simulink model "SF042A_HwAgSnsrls"  (R2013b)
settings: Solver=FixedStepDiscrete  SolverMode=SingleTasking  StartTime=0.0  StopTime=1  FixedStep=0.002  RelTol=1e-3
values from neighbouring files (symbols this model uses):
  ARCHGLBPRM_2MILLISEC_SEC_F32 = DataDict.Constant    [SF042A_HwAgSnsrls_DataDict.m]
  CORRDPINIONAGCON_CNT_U08 = DataDict.Constant    [SF042A_HwAgSnsrls_DataDict.m]
  FCENTROFFSCON_CNT_U08 = DataDict.Constant    [SF042A_HwAgSnsrls_DataDict.m]
  HwAgSnsrlsCorrdPinionAgHwConf = DataDict.Calibration    [SF042A_HwAgSnsrls_DataDict.m]
  HwAgSnsrlsFCentrHwConf = DataDict.Calibration    [SF042A_HwAgSnsrls_DataDict.m]
  HwAgSnsrlsSmotngCoeff = DataDict.Calibration    [SF042A_HwAgSnsrls_DataDict.m]
  HwAgSnsrlsSmotngStepThd = DataDict.Calibration    [SF042A_HwAgSnsrls_DataDict.m]
  HwAgSnsrlsStordPinionConf = DataDict.Calibration    [SF042A_HwAgSnsrls_DataDict.m]
  HwAgSnsrlsStordPinionConfThd = DataDict.Calibration    [SF042A_HwAgSnsrls_DataDict.m]
  HwAgSnsrlsVehDynDifThd = DataDict.Calibration    [SF042A_HwAgSnsrls_DataDict.m]
  HwAgSnsrlsVehDynHwConf = DataDict.Calibration    [SF042A_HwAgSnsrls_DataDict.m]
  HwAgSnsrlsVehDynMotVelThd = DataDict.Calibration    [SF042A_HwAgSnsrls_DataDict.m]
  HwAgSnsrlsVehDynPinionTqThd = DataDict.Calibration    [SF042A_HwAgSnsrls_DataDict.m]
  HwAgSnsrlsVehDynTmr1Thd = DataDict.Calibration    [SF042A_HwAgSnsrls_DataDict.m]
  HwAgSnsrlsVehDynTmr2Thd = DataDict.Calibration    [SF042A_HwAgSnsrls_DataDict.m]
  HwAgSnsrlsVehDynVehSpdThd = DataDict.Calibration    [SF042A_HwAgSnsrls_DataDict.m]
  HwAgSnsrlsVehDynYawRateThd = DataDict.Calibration    [SF042A_HwAgSnsrls_DataDict.m]
  HwAgSnsrlsWhlFrqThd = DataDict.Calibration    [SF042A_HwAgSnsrls_DataDict.m]
  HwAgSnsrlsWhlSpdHwAgCoeff1 = DataDict.Calibration    [SF042A_HwAgSnsrls_DataDict.m]
  HwAgSnsrlsWhlSpdHwAgCoeff2 = DataDict.Calibration    [SF042A_HwAgSnsrls_DataDict.m]
  HwAgSnsrlsWhlSpdHwAgThd = DataDict.Calibration    [SF042A_HwAgSnsrls_DataDict.m]
  HwAgSnsrlsWhlSpdHwConf = DataDict.Calibration    [SF042A_HwAgSnsrls_DataDict.m]
  HwAgSnsrlsWhlSpdRatThd = DataDict.Calibration    [SF042A_HwAgSnsrls_DataDict.m]
  HwAgSnsrlsWhlSpdTmrThd = DataDict.Calibration    [SF042A_HwAgSnsrls_DataDict.m]
  HwAgSnsrlsWhlSpdVehSpdThd = DataDict.Calibration    [SF042A_HwAgSnsrls_DataDict.m]
  LASTPOSNCON_CNT_U08 = DataDict.Constant    [SF042A_HwAgSnsrls_DataDict.m]
  MILLISECTO100MICROSEC_ULS_U32 = DataDict.Constant    [SF042A_HwAgSnsrls_DataDict.m]
  SysGlbPrmSysKineRat = DataDict.ImprtdCal    [SF042A_HwAgSnsrls_DataDict.m]
  SysGlbPrmSysTqRat = DataDict.ImprtdCal    [SF042A_HwAgSnsrls_DataDict.m]
  VEHDYNCON_CNT_U08 = DataDict.Constant    [SF042A_HwAgSnsrls_DataDict.m]
  WHLSPDCON_CNT_U08 = DataDict.Constant    [SF042A_HwAgSnsrls_DataDict.m]
undefined symbols (not defined in the file or in its folder): NtcNr1, SigQlfr1
libraries: NxtrAbslt x11, Fil x8, NxtrLim x4, simulink x3, NxtrNvM x1, FixdToFloat x1
(part 2 of 6)

== system SF042A_HwAgSnsrls/HwAgSnsrls/HwAgSnsrlsInit1/FiltersInit ==
  CopyRight2 : Subsystem  Description=|  mask(Copyright Information){none=on}
      | Copyright info block.                                               
      |                                                                     
      | Place copyright information at the top of every subsystem in design.
      mask prompts: none "No parameters"
      mask help: Place copyright information at the top of every subsystem in design.
      mask Display:
      | NxtrConf = 'Nexteer Confidential';
      | 
      | sys = bdroot; %handle for the current model ("system")
      | first = get_param(sys,'Created');
      | if(isempty(first))
      |     first = datestr(now,'yyyy');
      | else
      |     first = first(end-3:end);  %year is last four digits
      | end
      | 
      | last = get_param(sys,'LastModifiedDate');
      | if isempty(last)
      |     last = datestr(now,'yyyy');
      | else
      |     last = last(end-3:end);
      | end
      | 
      | if strcmp(first,last)
      |     fprintf('%s -- Copyright %s Nexteer',NxtrConf,first)
      | else
      |     fprintf('%s -- %s%s- %s Nexteer',NxtrConf,char(169),first,last)
      | end
  PinionTqFilInit : Fil/FilLpInit  Ic=0  Ts=ARCHGLBPRM_2MILLISEC_SEC_F32  Freq=HwAgSnsrlsPinionTqFilFrq  StVar=PinionTqFil
  RelHwAgFil1Init : Fil/FilLpInit  Ic=0  Ts=ARCHGLBPRM_2MILLISEC_SEC_F32  Freq=HwAgSnsrlsRelHwAgFil1Frq  StVar=RelHwAgFil1
  RelHwAgFil2Init : Fil/FilLpInit  Ic=0  Ts=ARCHGLBPRM_2MILLISEC_SEC_F32  Freq=HwAgSnsrlsRelHwAgFil2Frq  StVar=RelHwAgFil2
  YawRateFilInit : Fil/FilLpInit  Ic=0  Ts=ARCHGLBPRM_2MILLISEC_SEC_F32  Freq=HwAgSnsrlsYawRateFilFrq  StVar=YawRateFil

== system SF042A_HwAgSnsrls/HwAgSnsrls/HwAgSnsrlsInit1/GetNtcQlfrSts ==
  NtcNr : Inport
  CopyRight2 : Subsystem  Description=|  mask(Copyright Information){none=on}
      | Copyright info block.                                               
      |                                                                     
      | Place copyright information at the top of every subsystem in design.
      mask prompts: none "No parameters"
      mask help: Place copyright information at the top of every subsystem in design.
      mask Display:
      | NxtrConf = 'Nexteer Confidential';
      | 
      | sys = bdroot; %handle for the current model ("system")
      | first = get_param(sys,'Created');
      | first = first(end-3:end);  %year is last four digits
      | 
      | last = get_param(sys,'LastModifiedDate');
      | if isempty(last)
      |     last = datestr(now,'yyyy');
      | else
      |     last = last(end-3:end);
      | end
      | 
      | if strcmp(first,last)
      |     fprintf('%s -- Copyright %s Nexteer',NxtrConf,first)
      | else
      |     fprintf('%s -- %s%s- %s Nexteer',NxtrConf,char(169),first,last)
      | end
  Data Store Read : DataStoreRead  DataStoreName=NtcQlfr
  Terminator : Terminator
  NtcQlfr : Outport
  wires:
  Data Store Read/1 -> NtcQlfr/1
  NtcNr/1 -> Terminator/1

== system SF042A_HwAgSnsrls/HwAgSnsrls/HwAgSnsrlsInit1/GetRefTmr100MicroSec32bit ==
  note: Created Aug 18, 2015
      | Modified Oct 21, 2015
      | Modified Oct 30, 2015
      | Kevin Derry
  note: GetRefTmr100MicroSec32bit
  note: Wrap-to-zero
  note: counts
  note: microseconds
  note: seconds
  note: 1 count = 100 uSec
  CopyRight2 : Subsystem  Description=|  mask(Copyright Information){none=on}
      | Copyright info block.                                               
      |                                                                     
      | Place copyright information at the top of every subsystem in design.
      mask prompts: none "No parameters"
      mask help: Place copyright information at the top of every subsystem in design.
      mask Display:
      | NxtrConf = 'Nexteer Confidential';
      | 
      | sys = bdroot; %handle for the current model ("system")
      | first = get_param(sys,'Created');
      | if(isempty(first))
      |     first = datestr(now,'yyyy');
      | else
      |     first = first(end-3:end);  %year is last four digits
      | end
      | 
      | last = get_param(sys,'LastModifiedDate');
      | if isempty(last)
      |     last = datestr(now,'yyyy');
      | else
      |     last = last(end-3:end);
      | end
      | 
      | if strcmp(first,last)
      |     fprintf('%s -- Copyright %s Nexteer',NxtrConf,first)
      | else
      |     fprintf('%s -- %s%s- %s Nexteer',NxtrConf,char(169),first,last)
      | end
  Count per uSec : Constant  Value=0.01
  Data Store Read1 : DataStoreRead  DataStoreName=SimnTi
  Data Type Conversion1 : DataTypeConversion  OutDataTypeStr=uint32
  Divide1 : Product  Inputs=**
  Divide2 : Product  Inputs=*/
  Max Counts : Constant  Value=2^32-1
  Product1 : Product
  Product2 : Product
  Rounding : Rounding
  Subtract1 : Sum  Inputs=+-
  uSec per Sec : Constant  Value=1000000
  RefTmr : Outport
  wires:
  Data Store Read1/1 -> Product1/1
  Data Type Conversion1/1 -> RefTmr/1
  uSec per Sec/1 -> Product1/2
  Count per uSec/1 -> Divide1/2
  Product1/1 -> Divide1/1
  Divide1/1 -> Subtract1/1, Divide2/1
  Max Counts/1 -> Product2/2, Divide2/2
  Divide2/1 -> Rounding/1
  Rounding/1 -> Product2/1
  Subtract1/1 -> Data Type Conversion1/1
  Product2/1 -> Subtract1/2

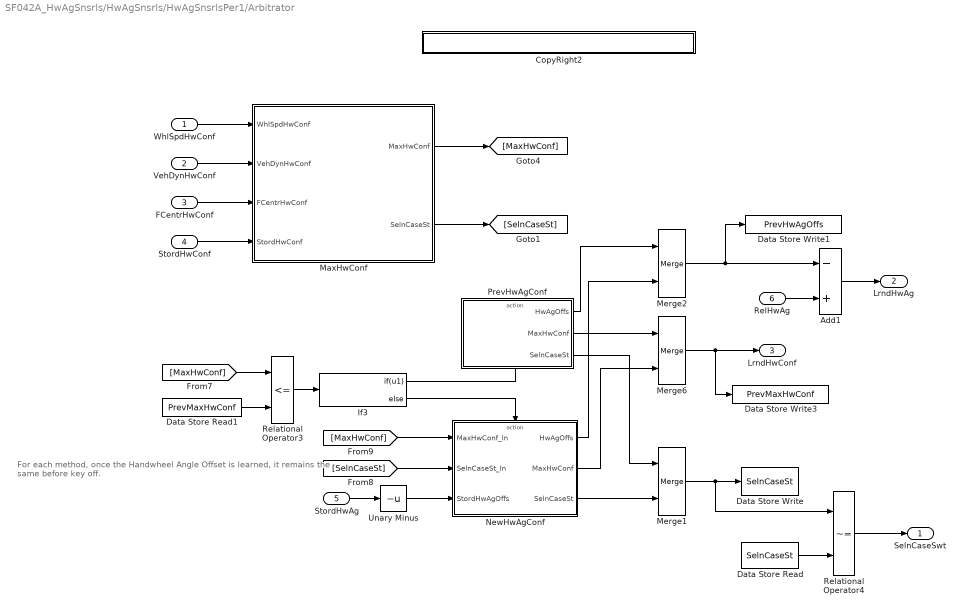
== system SF042A_HwAgSnsrls/HwAgSnsrls/HwAgSnsrlsPer1/Arbitrator ==
  note: For each method, once the Handwheel Angle Offset is learned, it remains the
      | same before key off.
  WhlSpdHwConf : Inport
  VehDynHwConf : Inport  Port=2
  FCentrHwConf : Inport  Port=3
  StordHwConf : Inport  Port=4
  StordHwAg : Inport  Port=5
  RelHwAg : Inport  Port=6
  Add1 : Sum  RequirementInfo="{'linktype_rmi_doors' '00012961 (/E-STEER Core/SubSystem Specifications/Application Functions - EA4/SF042A Handwheel Angle Sensorless)' '#SF042A_91' 'true' 'REQ:  SF042A_91' '' } %GIDa_1ccd16d5_cbcc_41e9_85e2_2e3643f02b11"  Inputs=-+
  CopyRight2 : Subsystem  Description=|  mask(Copyright Information){none=on}
      | Copyright info block.                                               
      |                                                                     
      | Place copyright information at the top of every subsystem in design.
      mask prompts: none "No parameters"
      mask help: Place copyright information at the top of every subsystem in design.
      mask Display:
      | NxtrConf = 'Nexteer Confidential';
      | 
      | sys = bdroot; %handle for the current model ("system")
      | first = get_param(sys,'Created');
      | if(isempty(first))
      |     first = datestr(now,'yyyy');
      | else
      |     first = first(end-3:end);  %year is last four digits
      | end
      | 
      | last = get_param(sys,'LastModifiedDate');
      | if isempty(last)
      |     last = datestr(now,'yyyy');
      | else
      |     last = last(end-3:end);
      | end
      | 
      | if strcmp(first,last)
      |     fprintf('%s -- Copyright %s Nexteer',NxtrConf,first)
      | else
      |     fprintf('%s -- %s%s- %s Nexteer',NxtrConf,char(169),first,last)
      | end
  Data Store Read : DataStoreRead  Priority=1  DataStoreName=SelnCaseSt
  Data Store Read1 : DataStoreRead  RequirementInfo={} %GIDa_f23f8d3d_c4da_4f79_957d_263e33d41729  DataStoreName=PrevMaxHwConf
  Data Store Write : DataStoreWrite  Priority=2  DataStoreName=SelnCaseSt
  Data Store Write1 : DataStoreWrite  DataStoreName=PrevHwAgOffs
  Data Store Write3 : DataStoreWrite  DataStoreName=PrevMaxHwConf
  If3 : If  RequirementInfo={'linktype_rmi_doors' '00012961 (/E-STEER Core/SubSystem Specifications/Application Functions - EA4/SF042A Handwheel Angle Sensorless)' '#SF042A_80' 'true' 'REQ:SF042A_80' '' ; 'linktype_rmi_doors' '00012961 (/E-STEER Core/SubSystem Specifications/Application Functions - EA4/SF042A Handwheel Angle Sensorless)' '#SF042A_90' 'true' 'REQ:SF042A_90' '' } %GIDa_130cdf60_6fef_48e9_8b09_d21ec738d534  IfExpression=u1
  MaxHwConf : Subsystem  RequirementInfo={'linktype_rmi_doors' '00012961 (/E-STEER Core/SubSystem Specifications/Application Functions - EA4/SF042A Handwheel Angle Sensorless)' '#SF042A_80' 'true' 'REQ:SF042A_80' '' } %GIDa_e5157a28_4abb_4275_9ef4_fab061bcf0ff
  Merge1 : Merge  RequirementInfo={'linktype_rmi_doors' '00012961 (/E-STEER Core/SubSystem Specifications/Application Functions - EA4/SF042A Handwheel Angle Sensorless)' '#SF042A_90' 'true' 'REQ:SF042A_90' '' ; 'linktype_rmi_doors' '00012961 (/E-STEER Core/SubSystem Specifications/Application Functions - EA4/SF042A Handwheel Angle Sensorless)' '#SF042A_80' 'true' 'REQ:SF042A_80' '' } %GIDa_5b272a3b_1995_4619_bc08_9d470fec44f3
  Merge2 : Merge  RequirementInfo={'linktype_rmi_doors' '00012961 (/E-STEER Core/SubSystem Specifications/Application Functions - EA4/SF042A Handwheel Angle Sensorless)' '#SF042A_90' 'true' 'REQ:SF042A_90' '' ; 'linktype_rmi_doors' '00012961 (/E-STEER Core/SubSystem Specifications/Application Functions - EA4/SF042A Handwheel Angle Sensorless)' '#SF042A_80' 'true' 'REQ:SF042A_80' '' } %GIDa_c0f8c842_a58b_4714_b1d4_ec4b723ea5b6
  Merge6 : Merge  RequirementInfo={'linktype_rmi_doors' '00012961 (/E-STEER Core/SubSystem Specifications/Application Functions - EA4/SF042A Handwheel Angle Sensorless)' '#SF042A_90' 'true' 'REQ:SF042A_90' '' ; 'linktype_rmi_doors' '00012961 (/E-STEER Core/SubSystem Specifications/Application Functions - EA4/SF042A Handwheel Angle Sensorless)' '#SF042A_80' 'true' 'REQ:SF042A_80' '' } %GIDa_12b5e5e2_09a6_4992_9385_b86d5bcd82fa
  NewHwAgConf : Subsystem  RequirementInfo={'linktype_rmi_doors' '00012961 (/E-STEER Core/SubSystem Specifications/Application Functions - EA4/SF042A Handwheel Angle Sensorless)' '#SF042A_80' 'true' 'REQ:SF042A_80' '' } %GIDa_82674b30_ff3b_4424_92dc_60f07d4aa3b1  TreatAsAtomicUnit=on
  PrevHwAgConf : Subsystem  RequirementInfo={'linktype_rmi_doors' '00012961 (/E-STEER Core/SubSystem Specifications/Application Functions - EA4/SF042A Handwheel Angle Sensorless)' '#SF042A_90' 'true' 'REQ:SF042A_90' '' } %GIDa_34576ddf_b2ec_4043_bac4_f5bd2e7329f0  TreatAsAtomicUnit=on
  Relational Operator3 : RelationalOperator  RequirementInfo={'linktype_rmi_doors' '00012961 (/E-STEER Core/SubSystem Specifications/Application Functions - EA4/SF042A Handwheel Angle Sensorless)' '#SF042A_80' 'true' 'REQ:SF042A_80' '' ; 'linktype_rmi_doors' '00012961 (/E-STEER Core/SubSystem Specifications/Application Functions - EA4/SF042A Handwheel Angle Sensorless)' '#SF042A_90' 'true' 'REQ:SF042A_90' '' } %GIDa_f55476d1_a2bc_48a5_a5ff_0b6ad56709cd  Operator=<=  OutDataTypeStr=boolean
  Relational Operator4 : RelationalOperator  RequirementInfo={'linktype_rmi_doors' '00012961 (/E-STEER Core/SubSystem Specifications/Application Functions - EA4/SF042A Handwheel Angle Sensorless)' '#SF042A_81' 'true' 'REQ: SF042A_81' '' } %GIDa_b2c97a21_2f99_417c_b86c_11bc5588197e  Operator=~=  OutDataTypeStr=boolean
  Unary Minus : UnaryMinus
  SelnCaseSwt : Outport
  LrndHwAg : Outport  Port=2
  LrndHwConf : Outport  Port=3
  wires:
  [MaxHwConf] -> Relational Operator3/1
  Data Store Read1/1 -> Relational Operator3/2
  Relational Operator3/1 -> If3/1
  If3/1 -> PrevHwAgConf/Action
  If3/2 -> NewHwAgConf/Action
  [SelnCaseSt] -> NewHwAgConf/2(SelnCaseSt_In)
  [MaxHwConf] -> NewHwAgConf/1(MaxHwConf_In)
  PrevHwAgConf/2(MaxHwConf) -> Merge6/1
  Merge6/1 -> Data Store Write3/1, LrndHwConf/1
  NewHwAgConf/2(MaxHwConf) -> Merge6/2
  StordHwAg/1 -> Unary Minus/1
  Unary Minus/1 -> NewHwAgConf/3(StordHwAgOffs)
  Merge2/1 -> Data Store Write1/1, Add1/1
  RelHwAg/1 -> Add1/2
  Add1/1 -> LrndHwAg/1
  WhlSpdHwConf/1 -> MaxHwConf/1(WhlSpdHwConf)
  VehDynHwConf/1 -> MaxHwConf/2(VehDynHwConf)
  FCentrHwConf/1 -> MaxHwConf/3(FCentrHwConf)
  StordHwConf/1 -> MaxHwConf/4(StordHwConf)
  MaxHwConf/1(MaxHwConf) -> [MaxHwConf]
  MaxHwConf/2(SelnCaseSt) -> [SelnCaseSt]
  Data Store Read/1 -> Relational Operator4/2
  Relational Operator4/1 -> SelnCaseSwt/1
  NewHwAgConf/3(SelnCaseSt) -> Merge1/2
  PrevHwAgConf/3(SelnCaseSt) -> Merge1/1
  Merge1/1 -> Data Store Write/1, Relational Operator4/1
  NewHwAgConf/1(HwAgOffs) -> Merge2/2
  PrevHwAgConf/1(HwAgOffs) -> Merge2/1

== system SF042A_HwAgSnsrls/HwAgSnsrls/HwAgSnsrlsPer1/Case Invalid ==
  Action Port : ActionPort  ActionType=else
  Constant= : Constant  Value=false  OutDataTypeStr=boolean
      settings: AttributesFormatString=%<OutDataTypeStr>
  Constant=1 : Constant  Value=0  OutDataTypeStr=single
      settings: AttributesFormatString=%<OutDataTypeStr>
  CopyRight2 : Subsystem  Description=|  mask(Copyright Information){none=on}
      | Copyright info block.                                               
      |                                                                     
      | Place copyright information at the top of every subsystem in design.
      mask prompts: none "No parameters"
      mask help: Place copyright information at the top of every subsystem in design.
      mask Display:
      | NxtrConf = 'Nexteer Confidential';
      | 
      | sys = bdroot; %handle for the current model ("system")
      | first = get_param(sys,'Created');
      | if(isempty(first))
      |     first = datestr(now,'yyyy');
      | else
      |     first = first(end-3:end);  %year is last four digits
      | end
      | 
      | last = get_param(sys,'LastModifiedDate');
      | if isempty(last)
      |     last = datestr(now,'yyyy');
      | else
      |     last = last(end-3:end);
      | end
      | 
      | if strcmp(first,last)
      |     fprintf('%s -- Copyright %s Nexteer',NxtrConf,first)
      | else
      |     fprintf('%s -- %s%s- %s Nexteer',NxtrConf,char(169),first,last)
      | end
  StordPinionAg : Outport
  StordPinionAgVld : Outport  Port=2
  wires:
  Constant=1/1 -> StordPinionAg/1
  Constant=/1 -> StordPinionAgVld/1

== system SF042A_HwAgSnsrls/HwAgSnsrls/HwAgSnsrlsPer1/Case Valid ==
  PinionAg : Inport
  Action Port : ActionPort  ActionType=then
  Constant= : Constant  Value=true  OutDataTypeStr=boolean
      settings: AttributesFormatString=%<OutDataTypeStr>
  CopyRight2 : Subsystem  Description=|  mask(Copyright Information){none=on}
      | Copyright info block.                                               
      |                                                                     
      | Place copyright information at the top of every subsystem in design.
      mask prompts: none "No parameters"
      mask help: Place copyright information at the top of every subsystem in design.
      mask Display:
      | NxtrConf = 'Nexteer Confidential';
      | 
      | sys = bdroot; %handle for the current model ("system")
      | first = get_param(sys,'Created');
      | if(isempty(first))
      |     first = datestr(now,'yyyy');
      | else
      |     first = first(end-3:end);  %year is last four digits
      | end
      | 
      | last = get_param(sys,'LastModifiedDate');
      | if isempty(last)
      |     last = datestr(now,'yyyy');
      | else
      |     last = last(end-3:end);
      | end
      | 
      | if strcmp(first,last)
      |     fprintf('%s -- Copyright %s Nexteer',NxtrConf,first)
      | else
      |     fprintf('%s -- %s%s- %s Nexteer',NxtrConf,char(169),first,last)
      | end
  StordPinionAg : Outport
  StordPinionAgVld : Outport  Port=2
  wires:
  Constant=/1 -> StordPinionAgVld/1
  PinionAg/1 -> StordPinionAg/1

== system SF042A_HwAgSnsrls/HwAgSnsrls/HwAgSnsrlsPer1/CopyRight2 ==

== system SF042A_HwAgSnsrls/HwAgSnsrls/HwAgSnsrlsPer1/CorrdPinionAg ==
  RelHwAg : Inport  RequirementInfo="{'linktype_rmi_doors' '00012961 (/E-STEER Core/SubSystem Specifications/Application Functions - EA4/SF042A Handwheel Angle Sensorless)' '#SF042A_98' 'true' 'REQ:  SF042A_98' '' } %GIDa_31b88bd3_f859_4e44_9356_ad3d0ab6ee77"
  PinionAg : Inport  RequirementInfo="{'linktype_rmi_doors' '00012961 (/E-STEER Core/SubSystem Specifications/Application Functions - EA4/SF042A Handwheel Angle Sensorless)' '#SF042A_98' 'true' 'REQ:  SF042A_98' '' } %GIDa_f824aa00_2535_4d02_9f51_7b39f985e134"  Port=2
  Action Port : ActionPort  ActionType=then
  Add : Sum  RequirementInfo="{'linktype_rmi_doors' '00012961 (/E-STEER Core/SubSystem Specifications/Application Functions - EA4/SF042A Handwheel Angle Sensorless)' '#SF042A_98' 'true' 'REQ:  SF042A_98' '' } %GIDa_c56c61bc_fb80_4014_afb5_ca03be690c09"  Inputs=+-
  Constant1 : Constant  RequirementInfo="{'linktype_rmi_doors' '00012961 (/E-STEER Core/SubSystem Specifications/Application Functions - EA4/SF042A Handwheel Angle Sensorless)' '#SF042A_36' 'true' 'REQ: SF042A_36' '' ; 'linktype_rmi_doors' '00012961 (/E-STEER Core/SubSystem Specifications/Application Functions - EA4/SF042A Handwheel Angle Sensorless)' '#SF042A_72' 'true' 'REQ: SF042A_72' '' ; 'linktype_rmi_doors' '00012961 (/E-STEER Core/SubSystem Specifications/Application Functions - EA4/SF042A Handwheel Angle Sensorless)' '#SF042A_97' 'true' 'REQ:  SF042A_97' '' } %GIDa_313b0f8b_6f5e_4bea_a70b_4ca4793cbdaf"  Value=HwAgSnsrlsCorrdPinionAgHwConf
  CopyRight2 : Subsystem  Description=|  mask(Copyright Information){none=on}
      | Copyright info block.                                               
      |                                                                     
      | Place copyright information at the top of every subsystem in design.
      mask prompts: none "No parameters"
      mask help: Place copyright information at the top of every subsystem in design.
      mask Display:
      | NxtrConf = 'Nexteer Confidential';
      | 
      | sys = bdroot; %handle for the current model ("system")
      | first = get_param(sys,'Created');
      | if(isempty(first))
      |     first = datestr(now,'yyyy');
      | else
      |     first = first(end-3:end);  %year is last four digits
      | end
      | 
      | last = get_param(sys,'LastModifiedDate');
      | if isempty(last)
      |     last = datestr(now,'yyyy');
      | else
      |     last = last(end-3:end);
      | end
      | 
      | if strcmp(first,last)
      |     fprintf('%s -- Copyright %s Nexteer',NxtrConf,first)
      | else
      |     fprintf('%s -- %s%s- %s Nexteer',NxtrConf,char(169),first,last)
      | end
  Data Store Write : DataStoreWrite  RequirementInfo="{'linktype_rmi_doors' '00012961 (/E-STEER Core/SubSystem Specifications/Application Functions - EA4/SF042A Handwheel Angle Sensorless)' '#SF042A_98' 'true' 'REQ:  SF042A_98' '' } %GIDa_aaa4bb20_1db1_4609_9705_85d738519f1e"  DataStoreName=CorrdPinionAgHwAgOffs
  Data Store Write1 : DataStoreWrite  RequirementInfo="{'linktype_rmi_doors' '00012961 (/E-STEER Core/SubSystem Specifications/Application Functions - EA4/SF042A Handwheel Angle Sensorless)' '#SF042A_97' 'true' 'REQ:  SF042A_97' '' } %GIDa_577a1d64_96be_43e6_9fbb_e826e63eee23"  DataStoreName=CorrdPinionAgHwConf
  wires:
  PinionAg/1 -> Add/2
  RelHwAg/1 -> Add/1
  Add/1 -> Data Store Write/1
  Constant1/1 -> Data Store Write1/1

== system SF042A_HwAgSnsrls/HwAgSnsrls/HwAgSnsrlsPer1/FCentr ==
  note: The PIM, FCentrHwAgOffs is removed.
  RelHwAg : Inport
  CopyRight2 : Subsystem  Description=|  mask(Copyright Information){none=on}
      | Copyright info block.                                               
      |                                                                     
      | Place copyright information at the top of every subsystem in design.
      mask prompts: none "No parameters"
      mask help: Place copyright information at the top of every subsystem in design.
      mask Display:
      | NxtrConf = 'Nexteer Confidential';
      | 
      | sys = bdroot; %handle for the current model ("system")
      | first = get_param(sys,'Created');
      | if(isempty(first))
      |     first = datestr(now,'yyyy');
      | else
      |     first = first(end-3:end);  %year is last four digits
      | end
      | 
      | last = get_param(sys,'LastModifiedDate');
      | if isempty(last)
      |     last = datestr(now,'yyyy');
      | else
      |     last = last(end-3:end);
      | end
      | 
      | if strcmp(first,last)
      |     fprintf('%s -- Copyright %s Nexteer',NxtrConf,first)
      | else
      |     fprintf('%s -- %s%s- %s Nexteer',NxtrConf,char(169),first,last)
      | end
  Data Store Read : DataStoreRead  RequirementInfo={'linktype_rmi_doors' '00012961 (/E-STEER Core/SubSystem Specifications/Application Functions - EA4/SF042A Handwheel Angle Sensorless)' '#SF042A_69' 'true' 'REQ: SF042A_69' '' } %GIDa_d9fc31bd_981a_4521_8bfb_1cbcd5df897a  DataStoreName=FCentrHwAgEna
  Data Store Read2 : DataStoreRead  RequirementInfo={} %GIDa_b1a9383a_e8dc_4d4c_acd4_1f605043c14e  DataStoreName=FCentrHwConf
  If Action Subsystem : Subsystem  RequirementInfo={'linktype_rmi_doors' '00012961 (/E-STEER Core/SubSystem Specifications/Application Functions - EA4/SF042A Handwheel Angle Sensorless)' '#SF042A_69' 'true' 'REQ: SF042A_69' '' } %GIDa_0c6e52f5_96de_4168_82df_888846a07605  TreatAsAtomicUnit=on
  If1 : If  RequirementInfo={'linktype_rmi_doors' '00012961 (/E-STEER Core/SubSystem Specifications/Application Functions - EA4/SF042A Handwheel Angle Sensorless)' '#SF042A_69' 'true' 'REQ: SF042A_69' '' } %GIDa_c2855657_fed7_42d7_97d5_3e63716701f4  IfExpression=u1  ShowElse=off
  FCentrHwConf : Outport
  wires:
  Data Store Read/1 -> If1/1
  RelHwAg/1 -> If Action Subsystem/1(RelHwAg)
  Data Store Read2/1 -> FCentrHwConf/1
  If1/1 -> If Action Subsystem/Action

== system SF042A_HwAgSnsrls/HwAgSnsrls/HwAgSnsrlsPer1/RelHwAgCalcn ==
  note: Actually, it is pinion coordinate. To be compatible with the other components,
      | use handwheel coordinate.
  MotAgCumvAlgndCrf : Inport  RequirementInfo={'linktype_rmi_doors' '00012961 (/E-STEER Core/SubSystem Specifications/Application Functions - EA4/SF042A Handwheel Angle Sensorless)' '#SF042A_66' 'true' 'REQ:SF042A_66' '' } %GIDa_7764a0ac_7688_44da_8f3d_34bc7a23cd33
  CmplncErrMotToPinion : Inport  Port=2
  MotAgCumvAlgndVld : Inport  Port=3
  Add : Sum  RequirementInfo={'linktype_rmi_doors' '00012961 (/E-STEER Core/SubSystem Specifications/Application Functions - EA4/SF042A Handwheel Angle Sensorless)' '#SF042A_66' 'true' 'REQ: SF042A_66' '' } %GIDa_6014d82f_05e8_41a9_bd83_46b327302849
  Add1 : Sum  RequirementInfo={'linktype_rmi_doors' '00012961 (/E-STEER Core/SubSystem Specifications/Application Functions - EA4/SF042A Handwheel Angle Sensorless)' '#SF042A_66' 'true' 'REQ: SF042A_66' '' ; 'linktype_rmi_doors' '00012961 (/E-STEER Core/SubSystem Specifications/Application Functions - EA4/SF042A Handwheel Angle Sensorless)' '#SF042A_66' 'true' 'REQ:SF042A_66' '' } %GIDa_16470bc5_c0d8_4493_8407_19d942f5b491  Inputs=+-
  Constant : Constant  RequirementInfo={'linktype_rmi_doors' '00012961 (/E-STEER Core/SubSystem Specifications/Application Functions - EA4/SF042A Handwheel Angle Sensorless)' '#SF042A_66' 'true' 'REQ: SF042A_66' '' } %GIDa_e1331208_1f56_4ad7_a69b_c0400a2e57c5  Value=SysGlbPrmSysKineRat
  CopyRight2 : Subsystem  Description=|  mask(Copyright Information){none=on}
      | Copyright info block.                                               
      |                                                                     
      | Place copyright information at the top of every subsystem in design.
      mask prompts: none "No parameters"
      mask help: Place copyright information at the top of every subsystem in design.
      mask Display:
      | NxtrConf = 'Nexteer Confidential';
      | 
      | sys = bdroot; %handle for the current model ("system")
      | first = get_param(sys,'Created');
      | if(isempty(first))
      |     first = datestr(now,'yyyy');
      | else
      |     first = first(end-3:end);  %year is last four digits
      | end
      | 
      | last = get_param(sys,'LastModifiedDate');
      | if isempty(last)
      |     last = datestr(now,'yyyy');
      | else
      |     last = last(end-3:end);
      | end
      | 
      | if strcmp(first,last)
      |     fprintf('%s -- Copyright %s Nexteer',NxtrConf,first)
      | else
      |     fprintf('%s -- %s%s- %s Nexteer',NxtrConf,char(169),first,last)
      | end
  Data Store Read2 : DataStoreRead  RequirementInfo={'linktype_rmi_doors' '00012961 (/E-STEER Core/SubSystem Specifications/Application Functions - EA4/SF042A Handwheel Angle Sensorless)' '#SF042A_66' 'true' 'REQ:SF042A_66' '' } %GIDa_ea549f90_b4c3_40d2_9e19_f23f1dab2180  DataStoreName=MotAgOffs
  Divide : Product  RequirementInfo={'linktype_rmi_doors' '00012961 (/E-STEER Core/SubSystem Specifications/Application Functions - EA4/SF042A Handwheel Angle Sensorless)' '#SF042A_66' 'true' 'REQ: SF042A_66' '' } %GIDa_1a03aa23_6b4b_44f2_97ee_7e85c475cbb9  Inputs=*/
  If : If  RequirementInfo={'linktype_rmi_doors' '00012961 (/E-STEER Core/SubSystem Specifications/Application Functions - EA4/SF042A Handwheel Angle Sensorless)' '#SF042A_66' 'true' 'REQ:SF042A_66' '' } %GIDa_26b64b67_062f_46d2_9cc1_7fd8b1c29971  IfExpression=u1
  LimStat_f32 : NxtrLim/LimStat_f32  RequirementInfo={'linktype_rmi_doors' '00012961 (/E-STEER Core/SubSystem Specifications/Application Functions - EA4/SF042A Handwheel Angle Sensorless)' '#SF042A_66' 'true' 'REQ: SF042A_66' '' } %GIDa_00db881e_0727_4441_9e0b_0f425127bd71  LoLim=HWAGLOLIM_HWDEG_F32  HiLim=HWAGHILIM_HWDEG_F32
      settings: AttributesFormatString=|
      | Low Limit: %<LoLim>
      | High Limit:%<HiLim>
  Merge : Merge  RequirementInfo={'linktype_rmi_doors' '00012961 (/E-STEER Core/SubSystem Specifications/Application Functions - EA4/SF042A Handwheel Angle Sensorless)' '#SF042A_66' 'true' 'REQ:SF042A_66' '' } %GIDa_ddede2be_b528_4cd0_a597_d7c5c66e8a8d
  Set to 0 : Subsystem  RequirementInfo={'linktype_rmi_doors' '00012961 (/E-STEER Core/SubSystem Specifications/Application Functions - EA4/SF042A Handwheel Angle Sensorless)' '#SF042A_66' 'true' 'REQ:SF042A_66' '' } %GIDa_21bc4451_8c70_4524_b3e6_24ec1d0ab393  TreatAsAtomicUnit=on
  UseMotAg : Subsystem  RequirementInfo={'linktype_rmi_doors' '00012961 (/E-STEER Core/SubSystem Specifications/Application Functions - EA4/SF042A Handwheel Angle Sensorless)' '#SF042A_66' 'true' 'REQ:SF042A_66' '' } %GIDa_3e176264_5296_4100_a678_93e3119ae127  TreatAsAtomicUnit=on
  RelHwAg : Outport
  wires:
  LimStat_f32/1 -> RelHwAg/1
  Add/1 -> LimStat_f32/1
  CmplncErrMotToPinion/1 -> Add/2
  Divide/1 -> Add/1
  Constant/1 -> Divide/2
  Add1/1 -> Divide/1
  MotAgCumvAlgndVld/1 -> If/1
  If/1 -> UseMotAg/Action
  If/2 -> Set to 0/Action
  MotAgCumvAlgndCrf/1 -> UseMotAg/1(MotAgCumvAlgndCrf)
  Set to 0/1(Out1) -> Merge/2
  UseMotAg/1(Out1) -> Merge/1
  Merge/1 -> Add1/1
  Data Store Read2/1 -> Add1/2

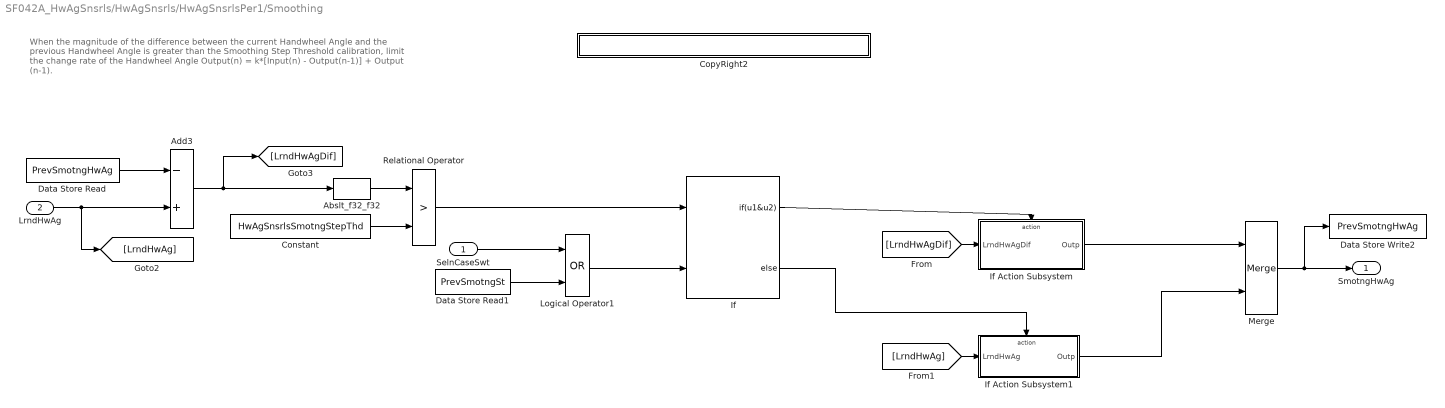
== system SF042A_HwAgSnsrls/HwAgSnsrls/HwAgSnsrlsPer1/Smoothing ==
  note: When the magnitude of the difference between the current Handwheel Angle and the
      |  previous Handwheel Angle is greater than the Smoothing Step Threshold calibration,
      |  limit the change rate of the Handwheel Angle
      |
      | 	Output(n) = k*[Input(n) - Output(n-1)] + Output (n-1).
  SelnCaseSwt : Inport  RequirementInfo={} %GIDa_c456bfc8_089b_4146_8336_dc474dc30222
  LrndHwAg : Inport  Port=2
  Abslt_f32_f32 : NxtrAbslt/Abslt_f32_f32  RequirementInfo={'linktype_rmi_doors' '00012961 (/E-STEER Core/SubSystem Specifications/Application Functions - EA4/SF042A Handwheel Angle Sensorless)' '#SF042A_89' 'true' 'REQ: SF042A_89' '' } %GIDa_50f05b6d_1032_4621_a61e_5ac84a4e8d74  SFunctionSpec=single y1 = Abslt_f32_f32(single u1)
      settings: AttributesFormatString=%<Name>
  Add3 : Sum  RequirementInfo={'linktype_rmi_doors' '00012961 (/E-STEER Core/SubSystem Specifications/Application Functions - EA4/SF042A Handwheel Angle Sensorless)' '#SF042A_89' 'true' 'REQ: SF042A_89' '' } %GIDa_4f76ac99_4af5_4a07_b8ac_e46f00bfc869  Inputs=-+
  Constant : Constant  RequirementInfo={'linktype_rmi_doors' '00012961 (/E-STEER Core/SubSystem Specifications/Application Functions - EA4/SF042A Handwheel Angle Sensorless)' '#SF042A_89' 'true' 'REQ: SF042A_89' '' } %GIDa_911e945b_6d72_4a85_ae06_3c37958c7dab  Value=HwAgSnsrlsSmotngStepThd
  CopyRight2 : Subsystem  Description=|  mask(Copyright Information){none=on}
      | Copyright info block.                                               
      |                                                                     
      | Place copyright information at the top of every subsystem in design.
      mask prompts: none "No parameters"
      mask help: Place copyright information at the top of every subsystem in design.
      mask Display:
      | NxtrConf = 'Nexteer Confidential';
      | 
      | sys = bdroot; %handle for the current model ("system")
      | first = get_param(sys,'Created');
      | if(isempty(first))
      |     first = datestr(now,'yyyy');
      | else
      |     first = first(end-3:end);  %year is last four digits
      | end
      | 
      | last = get_param(sys,'LastModifiedDate');
      | if isempty(last)
      |     last = datestr(now,'yyyy');
      | else
      |     last = last(end-3:end);
      | end
      | 
      | if strcmp(first,last)
      |     fprintf('%s -- Copyright %s Nexteer',NxtrConf,first)
      | else
      |     fprintf('%s -- %s%s- %s Nexteer',NxtrConf,char(169),first,last)
      | end
  Data Store Read : DataStoreRead  RequirementInfo={'linktype_rmi_doors' '00012961 (/E-STEER Core/SubSystem Specifications/Application Functions - EA4/SF042A Handwheel Angle Sensorless)' '#SF042A_89' 'true' 'REQ: SF042A_89' '' } %GIDa_10eb7aa0_da82_4d88_8196_8dc60e346702  DataStoreName=PrevSmotngHwAg
  Data Store Read1 : DataStoreRead  RequirementInfo={'linktype_rmi_doors' '00012961 (/E-STEER Core/SubSystem Specifications/Application Functions - EA4/SF042A Handwheel Angle Sensorless)' '#SF042A_89' 'true' 'REQ: SF042A_89' '' } %GIDa_b645a4ed_b50a_47e3_b1c4_760decad760d  DataStoreName=PrevSmotngSt
  Data Store Write2 : DataStoreWrite  DataStoreName=PrevSmotngHwAg
  If : If  RequirementInfo={'linktype_rmi_doors' '00012961 (/E-STEER Core/SubSystem Specifications/Application Functions - EA4/SF042A Handwheel Angle Sensorless)' '#SF042A_89' 'true' 'REQ: SF042A_89' '' } %GIDa_c366853c_b961_4a26_9337_2049d7eee2b6  NumInputs=2  IfExpression=u1&u2
  If Action Subsystem : Subsystem  RequirementInfo={'linktype_rmi_doors' '00012961 (/E-STEER Core/SubSystem Specifications/Application Functions - EA4/SF042A Handwheel Angle Sensorless)' '#SF042A_89' 'true' 'REQ: SF042A_89' '' } %GIDa_d017482d_d30a_47aa_a76a_a9d308daeccd  TreatAsAtomicUnit=on
  If Action Subsystem1 : Subsystem  RequirementInfo={'linktype_rmi_doors' '00012961 (/E-STEER Core/SubSystem Specifications/Application Functions - EA4/SF042A Handwheel Angle Sensorless)' '#SF042A_89' 'true' 'REQ: SF042A_89' '' } %GIDa_bfaf57c1_2252_42a2_b049_e0ec05601e26  TreatAsAtomicUnit=on
  Logical Operator1 : Logic  RequirementInfo={'linktype_rmi_doors' '00012961 (/E-STEER Core/SubSystem Specifications/Application Functions - EA4/SF042A Handwheel Angle Sensorless)' '#SF042A_89' 'true' 'REQ: SF042A_89' '' } %GIDa_fe9ffda4_60f0_4d80_8089_8bb31749b024  Operator=OR  AllPortsSameDT=off  OutDataTypeStr=boolean
  Merge : Merge  RequirementInfo={'linktype_rmi_doors' '00012961 (/E-STEER Core/SubSystem Specifications/Application Functions - EA4/SF042A Handwheel Angle Sensorless)' '#SF042A_89' 'true' 'REQ: SF042A_89' '' } %GIDa_77e904f2_7653_4624_9843_4cc4833fdfa4
  Relational Operator : RelationalOperator  RequirementInfo={'linktype_rmi_doors' '00012961 (/E-STEER Core/SubSystem Specifications/Application Functions - EA4/SF042A Handwheel Angle Sensorless)' '#SF042A_89' 'true' 'REQ: SF042A_89' '' } %GIDa_f84c138f_ed9c_48f5_944e_41b3fbac4839  Operator=>  OutDataTypeStr=boolean
  SmotngHwAg : Outport
  wires:
  [LrndHwAgDif] -> If Action Subsystem/1(LrndHwAgDif)
  [LrndHwAg] -> If Action Subsystem1/1(LrndHwAg)
  Add3/1 -> Abslt_f32_f32/1, [LrndHwAgDif]
  Relational Operator/1 -> If/1
  If/1 -> If Action Subsystem/Action
  If Action Subsystem1/1(Outp) -> Merge/2
  If Action Subsystem/1(Outp) -> Merge/1
  If/2 -> If Action Subsystem1/Action
  Merge/1 -> Data Store Write2/1, SmotngHwAg/1
  Data Store Read/1 -> Add3/1
  Constant/1 -> Relational Operator/2
  Abslt_f32_f32/1 -> Relational Operator/1
  Logical Operator1/1 -> If/2
  LrndHwAg/1 -> [LrndHwAg], Add3/2
  SelnCaseSwt/1 -> Logical Operator1/1
  Data Store Read1/1 -> Logical Operator1/2

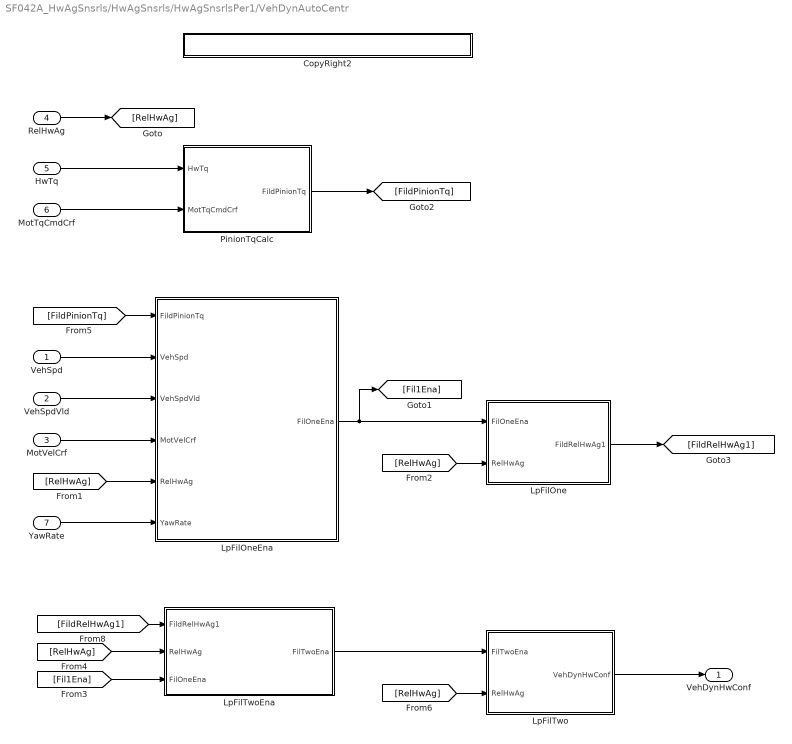
== system SF042A_HwAgSnsrls/HwAgSnsrls/HwAgSnsrlsPer1/VehDynAutoCentr ==
  VehSpd : Inport
  VehSpdVld : Inport  Port=2
  MotVelCrf : Inport  Port=3
  RelHwAg : Inport  Port=4
  HwTq : Inport  Port=5
  MotTqCmdCrf : Inport  Port=6
  YawRate : Inport  Port=7
  CopyRight2 : Subsystem  Description=|  mask(Copyright Information){none=on}
      | Copyright info block.                                               
      |                                                                     
      | Place copyright information at the top of every subsystem in design.
      mask prompts: none "No parameters"
      mask help: Place copyright information at the top of every subsystem in design.
      mask Display:
      | NxtrConf = 'Nexteer Confidential';
      | 
      | sys = bdroot; %handle for the current model ("system")
      | first = get_param(sys,'Created');
      | if(isempty(first))
      |     first = datestr(now,'yyyy');
      | else
      |     first = first(end-3:end);  %year is last four digits
      | end
      | 
      | last = get_param(sys,'LastModifiedDate');
      | if isempty(last)
      |     last = datestr(now,'yyyy');
      | else
      |     last = last(end-3:end);
      | end
      | 
      | if strcmp(first,last)
      |     fprintf('%s -- Copyright %s Nexteer',NxtrConf,first)
      | else
      |     fprintf('%s -- %s%s- %s Nexteer',NxtrConf,char(169),first,last)
      | end
  LpFilOne : Subsystem
  LpFilOneEna : Subsystem
  LpFilTwo : Subsystem
  LpFilTwoEna : Subsystem
  PinionTqCalc : Subsystem
  VehDynHwConf : Outport
  wires:
  YawRate/1 -> LpFilOneEna/6(YawRate)
  LpFilTwo/1(VehDynHwConf) -> VehDynHwConf/1
  PinionTqCalc/1(FildPinionTq) -> [FildPinionTq]
  MotTqCmdCrf/1 -> PinionTqCalc/2(MotTqCmdCrf)
  HwTq/1 -> PinionTqCalc/1(HwTq)
  [Fil1Ena] -> LpFilTwoEna/3(FilOneEna)
  LpFilTwoEna/1(FilTwoEna) -> LpFilTwo/1(FilTwoEna)
  [RelHwAg] -> LpFilTwoEna/2(RelHwAg)
  [FildRelHwAg1] -> LpFilTwoEna/1(FildRelHwAg1)
  [FildPinionTq] -> LpFilOneEna/1(FildPinionTq)
  MotVelCrf/1 -> LpFilOneEna/4(MotVelCrf)
  VehSpd/1 -> LpFilOneEna/2(VehSpd)
  VehSpdVld/1 -> LpFilOneEna/3(VehSpdVld)
  [RelHwAg] -> LpFilOneEna/5(RelHwAg)
  [RelHwAg] -> LpFilTwo/2(RelHwAg)
  LpFilOne/1(FildRelHwAg1) -> [FildRelHwAg1]
  LpFilOneEna/1(FilOneEna) -> LpFilOne/1(FilOneEna), [Fil1Ena]
  [RelHwAg] -> LpFilOne/2(RelHwAg)
  RelHwAg/1 -> [RelHwAg]

== system SF042A_HwAgSnsrls/HwAgSnsrls/HwAgSnsrlsPer1/WhlSpdAutoCentr ==
  WhlLeFrq : Inport
  WhlRiFrq : Inport  Port=2
  WhlFrqVld : Inport  Port=3
  VehSpd : Inport  Port=4
  RelHwAg : Inport  Port=5
  CopyRight2 : Subsystem  Description=|  mask(Copyright Information){none=on}
      | Copyright info block.                                               
      |                                                                     
      | Place copyright information at the top of every subsystem in design.
      mask prompts: none "No parameters"
      mask help: Place copyright information at the top of every subsystem in design.
      mask Display:
      | NxtrConf = 'Nexteer Confidential';
      | 
      | sys = bdroot; %handle for the current model ("system")
      | first = get_param(sys,'Created');
      | if(isempty(first))
      |     first = datestr(now,'yyyy');
      | else
      |     first = first(end-3:end);  %year is last four digits
      | end
      | 
      | last = get_param(sys,'LastModifiedDate');
      | if isempty(last)
      |     last = datestr(now,'yyyy');
      | else
      |     last = last(end-3:end);
      | end
      | 
      | if strcmp(first,last)
      |     fprintf('%s -- Copyright %s Nexteer',NxtrConf,first)
      | else
      |     fprintf('%s -- %s%s- %s Nexteer',NxtrConf,char(169),first,last)
      | end
  Data Store Write2 : DataStoreWrite  DataStoreName=dHwAgSnsrlsWhlSpdHwConf
  If : If  RequirementInfo={'linktype_rmi_doors' '00012961 (/E-STEER Core/SubSystem Specifications/Application Functions - EA4/SF042A Handwheel Angle Sensorless)' '#SF042A_85' 'true' 'REQ: SF042A_85' '' ; 'linktype_rmi_doors' '00012961 (/E-STEER Core/SubSystem Specifications/Application Functions - EA4/SF042A Handwheel Angle Sensorless)' '#SF042A_65' 'true' 'REQ: SF042A_65' '' } %GIDa_4d782368_1c4d_4e34_8907_6d5bd32dbf54  IfExpression=u1
  Merge1 : Merge  RequirementInfo={'linktype_rmi_doors' '00012961 (/E-STEER Core/SubSystem Specifications/Application Functions - EA4/SF042A Handwheel Angle Sensorless)' '#SF042A_85' 'true' 'REQ: SF042A_85' '' ; 'linktype_rmi_doors' '00012961 (/E-STEER Core/SubSystem Specifications/Application Functions - EA4/SF042A Handwheel Angle Sensorless)' '#SF042A_65' 'true' 'REQ: SF042A_65' '' } %GIDa_85c57ab6_9814_4a6a_82ac_ae8dc69b70dc
  WhlFrqNotVld : Subsystem  RequirementInfo={'linktype_rmi_doors' '00012961 (/E-STEER Core/SubSystem Specifications/Application Functions - EA4/SF042A Handwheel Angle Sensorless)' '#SF042A_85' 'true' 'REQ: SF042A_85' '' } %GIDa_d4cbccb1_a80b_4027_8410_34145e539bf7
  WhlSpd : Subsystem  RequirementInfo={'linktype_rmi_doors' '00012961 (/E-STEER Core/SubSystem Specifications/Application Functions - EA4/SF042A Handwheel Angle Sensorless)' '#SF042A_65' 'true' 'REQ: SF042A_65' '' } %GIDa_43a1e4ac_9069_478e_b50a_f6e2e6aa2af2
  WhlSpdHwConf : Outport
  wires:
  WhlFrqNotVld/1(WhlSpdHwConf) -> Merge1/2
  Merge1/1 -> WhlSpdHwConf/1, Data Store Write2/1
  If/2 -> WhlFrqNotVld/Action
  WhlSpd/1(WhlSpdHwConf) -> Merge1/1
  RelHwAg/1 -> WhlSpd/4(RelHwAg)
  WhlFrqVld/1 -> If/1
  If/1 -> WhlSpd/Action
  VehSpd/1 -> WhlSpd/3(VehSpd)
  WhlLeFrq/1 -> WhlSpd/1(WhlLeFrq)
  WhlRiFrq/1 -> WhlSpd/2(WhlRiFrq)

== system SF042A_HwAgSnsrls/HwAgSnsrls/RstSnsrlsHwCentr/CopyRight2 ==

== system SF042A_HwAgSnsrls/HwAgSnsrls/HwAgSnsrlsInit1/CaseNotValid/CopyRight2 ==

== system SF042A_HwAgSnsrls/HwAgSnsrls/HwAgSnsrlsInit1/CaseValid/CopyRight2 ==

== system SF042A_HwAgSnsrls/HwAgSnsrls/HwAgSnsrlsInit1/FiltersInit/CopyRight2 ==

== system SF042A_HwAgSnsrls/HwAgSnsrls/HwAgSnsrlsInit1/GetNtcQlfrSts/CopyRight2 ==

== system SF042A_HwAgSnsrls/HwAgSnsrls/HwAgSnsrlsInit1/GetRefTmr100MicroSec32bit/CopyRight2 ==

== system SF042A_HwAgSnsrls/HwAgSnsrls/HwAgSnsrlsPer1/Arbitrator/CopyRight2 ==

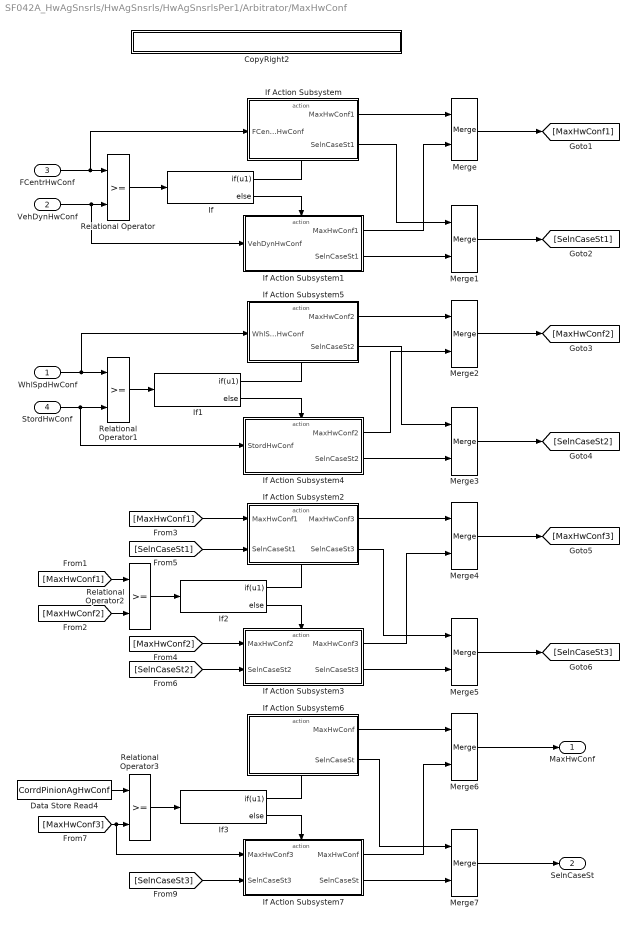
== system SF042A_HwAgSnsrls/HwAgSnsrls/HwAgSnsrlsPer1/Arbitrator/MaxHwConf ==
  WhlSpdHwConf : Inport
  VehDynHwConf : Inport  Port=2
  FCentrHwConf : Inport  Port=3
  StordHwConf : Inport  Port=4
  CopyRight2 : Subsystem  Description=|  mask(Copyright Information){none=on}
      | Copyright info block.                                               
      |                                                                     
      | Place copyright information at the top of every subsystem in design.
      mask prompts: none "No parameters"
      mask help: Place copyright information at the top of every subsystem in design.
      mask Display:
      | NxtrConf = 'Nexteer Confidential';
      | 
      | sys = bdroot; %handle for the current model ("system")
      | first = get_param(sys,'Created');
      | if(isempty(first))
      |     first = datestr(now,'yyyy');
      | else
      |     first = first(end-3:end);  %year is last four digits
      | end
      | 
      | last = get_param(sys,'LastModifiedDate');
      | if isempty(last)
      |     last = datestr(now,'yyyy');
      | else
      |     last = last(end-3:end);
      | end
      | 
      | if strcmp(first,last)
      |     fprintf('%s -- Copyright %s Nexteer',NxtrConf,first)
      | else
      |     fprintf('%s -- %s%s- %s Nexteer',NxtrConf,char(169),first,last)
      | end
  Data Store Read4 : DataStoreRead  RequirementInfo={} %GIDa_f50e7582_1734_4615_9728_09095c47a40c  DataStoreName=CorrdPinionAgHwConf
  If{,1..3} (4 alike) : If  IfExpression=u1
  If Action Subsystem : Subsystem  TreatAsAtomicUnit=on
  If Action Subsystem1 : Subsystem  TreatAsAtomicUnit=on
  If Action Subsystem2 : Subsystem  TreatAsAtomicUnit=on
  If Action Subsystem3 : Subsystem  TreatAsAtomicUnit=on
  If Action Subsystem4 : Subsystem  TreatAsAtomicUnit=on
  If Action Subsystem5 : Subsystem  TreatAsAtomicUnit=on
  If Action Subsystem6 : Subsystem  TreatAsAtomicUnit=on
  If Action Subsystem7 : Subsystem  TreatAsAtomicUnit=on
  Merge{,1..7} (8 alike) : Merge
  Relational Operator : RelationalOperator  OutDataTypeStr=boolean
  Relational Operator1 : RelationalOperator  OutDataTypeStr=boolean
  Relational Operator2 : RelationalOperator  OutDataTypeStr=boolean
  Relational Operator3 : RelationalOperator  RequirementInfo="{}  %GIDa_b9a0458f_f85a_4941_bd11_ccce90c2446f"  OutDataTypeStr=boolean
  MaxHwConf : Outport
  SelnCaseSt : Outport  Port=2
  wires:
  [SelnCaseSt1] -> If Action Subsystem2/2(SelnCaseSt1)
  Merge4/1 -> [MaxHwConf3]
  [MaxHwConf2] -> Relational Operator2/2
  [MaxHwConf1] -> Relational Operator2/1
  If1/1 -> If Action Subsystem5/Action
  Relational Operator1/1 -> If1/1
  If Action Subsystem4/1(MaxHwConf2) -> Merge2/2
  If Action Subsystem/1(MaxHwConf1) -> Merge/1
  If Action Subsystem4/2(SelnCaseSt2) -> Merge3/2
  If1/2 -> If Action Subsystem4/Action
  If Action Subsystem/2(SelnCaseSt1) -> Merge1/1
  If Action Subsystem1/2(SelnCaseSt1) -> Merge1/2
  If Action Subsystem5/1(MaxHwConf2) -> Merge2/1
  If Action Subsystem1/1(MaxHwConf1) -> Merge/2
  If Action Subsystem5/2(SelnCaseSt2) -> Merge3/1
  [SelnCaseSt2] -> If Action Subsystem3/2(SelnCaseSt2)
  Merge5/1 -> [SelnCaseSt3]
  If2/2 -> If Action Subsystem3/Action
  If Action Subsystem3/1(MaxHwConf3) -> Merge4/2
  If Action Subsystem3/2(SelnCaseSt3) -> Merge5/2
  [MaxHwConf2] -> If Action Subsystem3/1(MaxHwConf2)
  If Action Subsystem2/1(MaxHwConf3) -> Merge4/1
  If Action Subsystem2/2(SelnCaseSt3) -> Merge5/1
  If2/1 -> If Action Subsystem2/Action
  [MaxHwConf1] -> If Action Subsystem2/1(MaxHwConf1)
  WhlSpdHwConf/1 -> If Action Subsystem5/1(WhlSpdHwConf), Relational Operator1/1
  If/1 -> If Action Subsystem/Action
  Relational Operator/1 -> If/1
  Merge/1 -> [MaxHwConf1]
  Merge3/1 -> [SelnCaseSt2]
  Merge1/1 -> [SelnCaseSt1]
  Merge2/1 -> [MaxHwConf2]
  FCentrHwConf/1 -> If Action Subsystem/1(FCentrHwConf), Relational Operator/1
  VehDynHwConf/1 -> If Action Subsystem1/1(VehDynHwConf), Relational Operator/2
  Relational Operator2/1 -> If2/1
  If/2 -> If Action Subsystem1/Action
  StordHwConf/1 -> If Action Subsystem4/1(StordHwConf), Relational Operator1/2
  Relational Operator3/1 -> If3/1
  Data Store Read4/1 -> Relational Operator3/1
  If3/2 -> If Action Subsystem7/Action
  If3/1 -> If Action Subsystem6/Action
  If Action Subsystem6/1(MaxHwConf) -> Merge6/1
  If Action Subsystem6/2(SelnCaseSt) -> Merge7/1
  If Action Subsystem7/2(SelnCaseSt) -> Merge7/2
  If Action Subsystem7/1(MaxHwConf) -> Merge6/2
  [MaxHwConf3] -> If Action Subsystem7/1(MaxHwConf3), Relational Operator3/2
  [SelnCaseSt3] -> If Action Subsystem7/2(SelnCaseSt3)
  Merge6/1 -> MaxHwConf/1
  Merge7/1 -> SelnCaseSt/1

== system SF042A_HwAgSnsrls/HwAgSnsrls/HwAgSnsrlsPer1/Arbitrator/NewHwAgConf ==
  MaxHwConf_In : Inport
  SelnCaseSt_In : Inport  Port=2
  StordHwAgOffs : Inport  Port=3
  Action Port : ActionPort  ActionType=else
  CopyRight2 : Subsystem  Description=|  mask(Copyright Information){none=on}
      | Copyright info block.                                               
      |                                                                     
      | Place copyright information at the top of every subsystem in design.
      mask prompts: none "No parameters"
      mask help: Place copyright information at the top of every subsystem in design.
      mask Display:
      | NxtrConf = 'Nexteer Confidential';
      | 
      | sys = bdroot; %handle for the current model ("system")
      | first = get_param(sys,'Created');
      | if(isempty(first))
      |     first = datestr(now,'yyyy');
      | else
      |     first = first(end-3:end);  %year is last four digits
      | end
      | 
      | last = get_param(sys,'LastModifiedDate');
      | if isempty(last)
      |     last = datestr(now,'yyyy');
      | else
      |     last = last(end-3:end);
      | end
      | 
      | if strcmp(first,last)
      |     fprintf('%s -- Copyright %s Nexteer',NxtrConf,first)
      | else
      |     fprintf('%s -- %s%s- %s Nexteer',NxtrConf,char(169),first,last)
      | end
  HwAgOffsSeln : Subsystem  RequirementInfo={'linktype_rmi_doors' '00012961 (/E-STEER Core/SubSystem Specifications/Application Functions - EA4/SF042A Handwheel Angle Sensorless)' '#SF042A_80' 'true' 'REQ:SF042A_80' '' } %GIDa_8b62a219_2c88_469e_afe6_9be6d1caf2df
  HwAgOffs : Outport
  MaxHwConf : Outport  Port=2
  SelnCaseSt : Outport  Port=3
  wires:
  MaxHwConf_In/1 -> MaxHwConf/1
  SelnCaseSt_In/1 -> HwAgOffsSeln/2(SelnCaseSt), SelnCaseSt/1
  StordHwAgOffs/1 -> HwAgOffsSeln/1(StordHwAgOffs)
  HwAgOffsSeln/1(HwAgOffs) -> HwAgOffs/1

== system SF042A_HwAgSnsrls/HwAgSnsrls/HwAgSnsrlsPer1/Arbitrator/PrevHwAgConf ==
  Action Port : ActionPort  ActionType=then
  CopyRight2 : Subsystem  Description=|  mask(Copyright Information){none=on}
      | Copyright info block.                                               
      |                                                                     
      | Place copyright information at the top of every subsystem in design.
      mask prompts: none "No parameters"
      mask help: Place copyright information at the top of every subsystem in design.
      mask Display:
      | NxtrConf = 'Nexteer Confidential';
      | 
      | sys = bdroot; %handle for the current model ("system")
      | first = get_param(sys,'Created');
      | if(isempty(first))
      |     first = datestr(now,'yyyy');
      | else
      |     first = first(end-3:end);  %year is last four digits
      | end
      | 
      | last = get_param(sys,'LastModifiedDate');
      | if isempty(last)
      |     last = datestr(now,'yyyy');
      | else
      |     last = last(end-3:end);
      | end
      | 
      | if strcmp(first,last)
      |     fprintf('%s -- Copyright %s Nexteer',NxtrConf,first)
      | else
      |     fprintf('%s -- %s%s- %s Nexteer',NxtrConf,char(169),first,last)
      | end
  Data Store Read : DataStoreRead  DataStoreName=SelnCaseSt
  Data Store Read1 : DataStoreRead  DataStoreName=PrevMaxHwConf
  Data Store Read2 : DataStoreRead  DataStoreName=PrevHwAgOffs
  HwAgOffs : Outport
  MaxHwConf : Outport  Port=2
  SelnCaseSt : Outport  Port=3
  wires:
  Data Store Read1/1 -> MaxHwConf/1
  Data Store Read/1 -> SelnCaseSt/1
  Data Store Read2/1 -> HwAgOffs/1

== system SF042A_HwAgSnsrls/HwAgSnsrls/HwAgSnsrlsPer1/Case Invalid/CopyRight2 ==

== system SF042A_HwAgSnsrls/HwAgSnsrls/HwAgSnsrlsPer1/Case Valid/CopyRight2 ==

== system SF042A_HwAgSnsrls/HwAgSnsrls/HwAgSnsrlsPer1/CorrdPinionAg/CopyRight2 ==

== system SF042A_HwAgSnsrls/HwAgSnsrls/HwAgSnsrlsPer1/FCentr/CopyRight2 ==
